simulink model "Grading_System"  (R2018a)
settings: Solver=FixedStepDiscrete  StartTime=0.0  StopTime=10.0  RelTol=1e-3
settings Model: Creator=Moataz  LastModifiedBy=Moataz
settings OptimizationCC: DefaultParameterBehavior=Inlined  EnhancedBackFolding=on  PassReuseOutputArgsAs=Individual arguments  OptimizeBlockOrder=speed  DifferentSizesBufferReuse=on  OptimizationCustomize=off
settings DebuggingCC: ParameterTunabilityLossMsg=error
settings SFSimCC: MATLABDynamicMemAlloc=off
settings RTWCC: SystemTargetFile=ert.tlc  GenCodeOnly=on  TemplateMakefile=ert_default_tmf  GenerateReport=on  IncludeHyperlinkInReport=on  LaunchReport=on  GenerateTraceInfo=on  GenerateTraceReport=on  GenerateTraceReportSl=on  GenerateTraceReportSf=on  GenerateTraceReportEml=on
settings CodeAppCC: ForceParamTrailComments=on  IgnoreCustomStorageClasses=off  OperatorAnnotations=on  SimulinkDataObjDesc=on  SFDataObjDesc=on  InsertBlockDesc=on
settings ERTTargetCC: TargetLangStandard=C99 (ISO)  GenerateSampleERTMain=on  InlinedParameterPlacement=NonHierarchical  ERTCustomFileTemplate=example_file_process.tlc

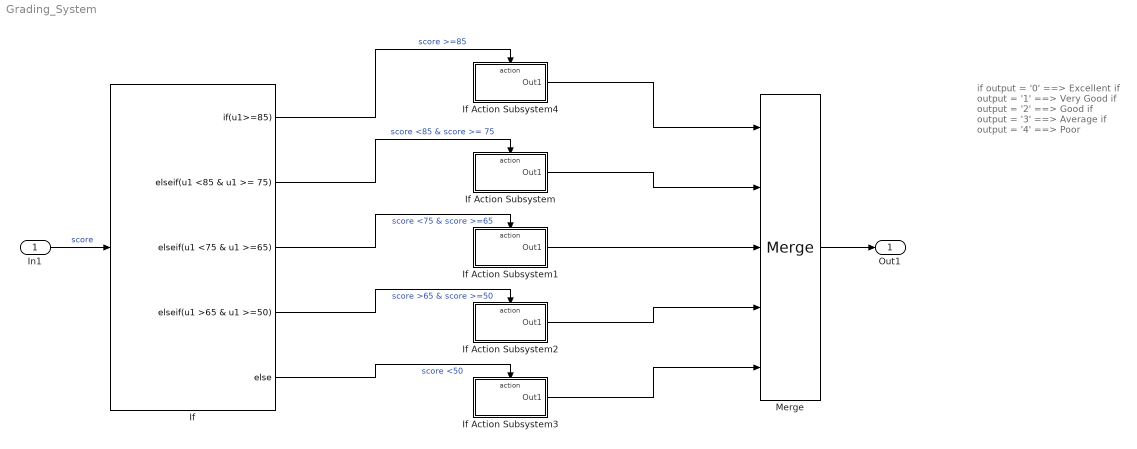
== system Grading_System ==
  note: if output = '0' ==> Excellent
      | if output = '1' ==> Very Good
      | if output = '2' ==> Good
      | if output = '3' ==> Average
      | if output = '4' ==> Poor
  In1 : Inport
  If : If  IfExpression=u1>=85  ElseIfExpressions=u1 <85 & u1 >= 75, u1 <75 & u1 >=65, u1 >65 & u1 >=50
  If Action Subsystem : Subsystem  TreatAsAtomicUnit=on
  If Action Subsystem1 : Subsystem  TreatAsAtomicUnit=on
  If Action Subsystem2 : Subsystem  TreatAsAtomicUnit=on
  If Action Subsystem3 : Subsystem  TreatAsAtomicUnit=on
  If Action Subsystem4 : Subsystem  TreatAsAtomicUnit=on
  Merge : Merge  Inputs=5
  Out1 : Outport
  wires:
  In1/1 -> If/1  "score"
  If/5 -> If Action Subsystem3/Action  "score <50"
  Merge/1 -> Out1/1
  If/4 -> If Action Subsystem2/Action  "score >65 & score >=50"
  If/3 -> If Action Subsystem1/Action  "score <75 & score >=65"
  If/2 -> If Action Subsystem/Action  "score <85 & score >= 75"
  If/1 -> If Action Subsystem4/Action  "score >=85"
  If Action Subsystem3/1(Out1) -> Merge/5
  If Action Subsystem2/1(Out1) -> Merge/4
  If Action Subsystem1/1(Out1) -> Merge/3
  If Action Subsystem/1(Out1) -> Merge/2
  If Action Subsystem4/1(Out1) -> Merge/1

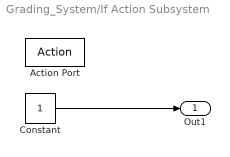
== system Grading_System/If Action Subsystem ==
  Action Port : ActionPort  ActionType=elseif
  Constant : Constant
  Out1 : Outport
  wires:
  Constant/1 -> Out1/1

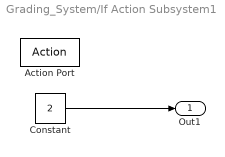
== system Grading_System/If Action Subsystem1 ==
  Action Port : ActionPort  ActionType=elseif
  Constant : Constant  Value=2
  Out1 : Outport
  wires:
  Constant/1 -> Out1/1

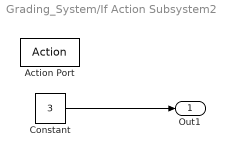
== system Grading_System/If Action Subsystem2 ==
  Action Port : ActionPort  ActionType=elseif
  Constant : Constant  Value=3
  Out1 : Outport
  wires:
  Constant/1 -> Out1/1

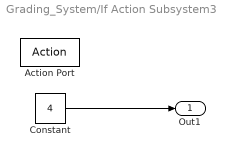
== system Grading_System/If Action Subsystem3 ==
  Action Port : ActionPort  ActionType=else
  Constant : Constant  Value=4
  Out1 : Outport
  wires:
  Constant/1 -> Out1/1

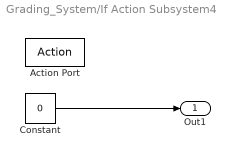
== system Grading_System/If Action Subsystem4 ==
  Action Port : ActionPort  ActionType=then
  Constant : Constant  Value=0
  Out1 : Outport
  wires:
  Constant/1 -> Out1/1
